simulink model "secorderpid2nd2015a"  (R2015a)
settings: Solver=ode23  SolverMode=SingleTasking  StartTime=0.0  StopTime=30  FixedStep=1e-3  MaxStep=5e-4  RelTol=5e-4
values from neighbouring files (symbols this model uses):
  b = [1 0]    [Example_IAE.mat]    (also in Exemple_1_disertacao.mat = 1; Exemple_3_disertacao.mat; example_result_gasearch.mat; example_result_gasearch_final.mat)
  C = [1  -1; -1  1]    [Example_IAE.mat]    (also in Exemple_1_disertacao.mat = 0.01; Exemple_3_disertacao.mat = [1  -0.9; -1  1]; example_result_gasearch.mat; example_result_gasearch_final.mat)
  d = [1 0]    [Example_IAE.mat]    (also in Exemple_1_disertacao.mat = 1; Exemple_3_disertacao.mat; example_result_gasearch.mat; example_result_gasearch_final.mat)
  dx0 = [0 0]    [Example_IAE.mat]    (also in Exemple_1_disertacao.mat; Exemple_3_disertacao.mat; example_result_gasearch.mat; example_result_gasearch_final.mat)
  K = [3  -2; -2  3]    [Example_IAE.mat]    (also in Exemple_1_disertacao.mat = 5; Exemple_3_disertacao.mat; example_result_gasearch.mat; example_result_gasearch_final.mat)
  M = [1  0; 0  1]    [Example_IAE.mat]    (also in Exemple_1_disertacao.mat = 1; Exemple_3_disertacao.mat; example_result_gasearch.mat; example_result_gasearch_final.mat)
  x0 = [0 0]    [Example_IAE.mat]    (also in Exemple_1_disertacao.mat; Exemple_3_disertacao.mat; example_result_gasearch.mat; example_result_gasearch_final.mat)
settings Model: SimulationMode=accelerator  Creator=Jose  LastModifiedBy=jhona
settings DataIOCC: SignalLoggingSaveFormat=ModelDataLogs
settings OptimizationCC: BlockReduction=off  BooleanDataType=off  ExpressionDepthLimit=2147483647  EfficientMapNaN2IntZero=off
settings DebuggingCC: SaveWithParameterizedLinksMsg=none  UnderspecifiedInitializationDetection=Classic  MergeDetectMultiDrivingBlocksExec=none  SignalResolutionControl=TryResolveAllWithWarning  MultiTaskDSMMsg=warning  MultiTaskCondExecSysMsg=none  StateNameClashWarn=warning
settings HardwareCC: TargetBitPerPointer=64  TargetLongLongMode=on  TargetIntDivRoundTo=Zero  TargetEndianess=LittleEndian  TargetWordSize=64  TargetHWDeviceType=MATLAB Host  ProdEqTarget=off
settings CodeAppCC: MaxIdLength=128
settings GRTTargetCC: CombineOutputUpdateFcns=off  GRTInterface=on

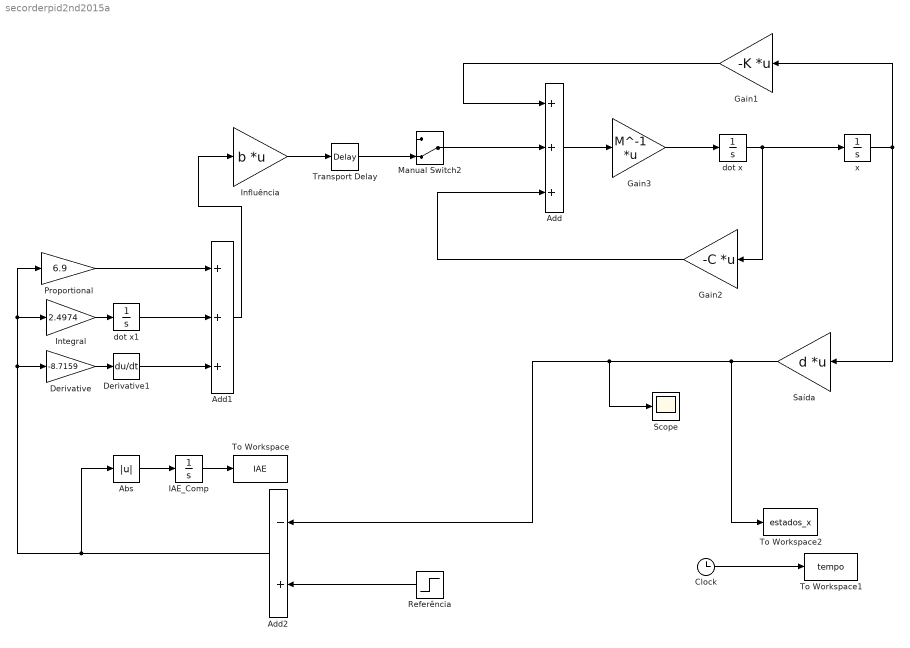
== system secorderpid2nd2015a ==
  Abs : Abs
  Add : Sum  Inputs=+++
  Add1 : Sum  Inputs=+++
  Add2 : Sum  Inputs=-+
  Clock : Clock
  Derivative : Gain  Gain=-8.7159
  Derivative1 : Derivative  CoefficientInTFapproximation=100
  Gain1 : Gain  Gain=-K  Multiplication=Matrix(K*u)
  Gain2 : Gain  Gain=-C  Multiplication=Matrix(K*u)
  Gain3 : Gain  Gain=M^-1  Multiplication=Matrix(K*u)
  IAE_Comp : Integrator
  Influência : Gain  Gain=b  Multiplication=Matrix(K*u)
  Integral : Gain  Gain=2.4974
  Manual Switch2 : ManualSwitch  CurrentSetting=0
  Proportional : Gain  Gain=6.9
  Referência : Step  SampleTime=0
  Saída : Gain  Gain=d  Multiplication=Matrix(K*u)
  Scope : Scope
      settings: TimeRange=25  MaxDataPoints=5000  SaveName=q  YMin=-2.75  YMax=2  SampleTime=-1  DataFormat=Array
  To Workspace : ToWorkspace  VariableName=IAE  SampleTime=-1
  To Workspace1 : ToWorkspace  VariableName=tempo  SampleTime=-1
  To Workspace2 : ToWorkspace  VariableName=estados_x  SampleTime=-1
  Transport Delay : TransportDelay  DelayTime=0.1  BufferSize=2048
  dot x : Integrator  InitialCondition=dx0
  dot x1 : Integrator
  x : Integrator  InitialCondition=x0
  wires:
  Gain1/1 -> Add/1
  Add/1 -> Gain3/1
  Gain3/1 -> dot x/1
  dot x/1 -> Gain2/1, x/1
  Gain2/1 -> Add/3
  Influência/1 -> Transport Delay/1
  Manual Switch2/1 -> Add/2
  Transport Delay/1 -> Manual Switch2/2
  Proportional/1 -> Add1/1
  Integral/1 -> dot x1/1
  dot x1/1 -> Add1/2
  Derivative1/1 -> Add1/3
  Derivative/1 -> Derivative1/1
  Referência/1 -> Add2/2
  Add1/1 -> Influência/1
  Add2/1 -> Abs/1, Proportional/1, Integral/1, Derivative/1
  Abs/1 -> IAE_Comp/1
  IAE_Comp/1 -> To Workspace/1
  Clock/1 -> To Workspace1/1
  x/1 -> Saída/1, Gain1/1
  Saída/1 -> To Workspace2/1, Scope/1, Add2/1
